simulink model "model_3_2018b"  (R2018b)
settings: Solver=VariableStepAuto  StartTime=0.0  StopTime=5  RelTol=1e-3  AbsTol=1e-3  EnableMultiTasking=on
undefined symbols (not defined in the file or in its folder): B, J, joints_traj, Kd1, Kd2, Ki1, Ki2, Km, Kp1, Kp2, max_v, r, Ra, radius, X, Y, Z
libraries: sm_lib x28, nesl_utility x17, simulink x3
(part 2 of 2)

== matlab function model_3_2018b/MATLAB Function ==
  data: u input; y output
function y = fcn(u)
y = norm(u)^2;
